simulink model "purePursuit"  (R2021b)
settings: Solver=VariableStepAuto  StartTime=0.0  StopTime=250  RelTol=1e-3
model workspace (MAT data in the model file):
  dg = 0.2
settings Model: Creator=ferna  LastModifiedBy=ferna

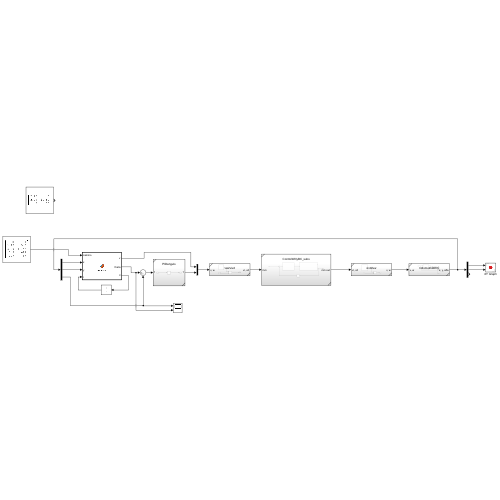
[thumbnail: Simulink's stored preview of the top-level diagram]
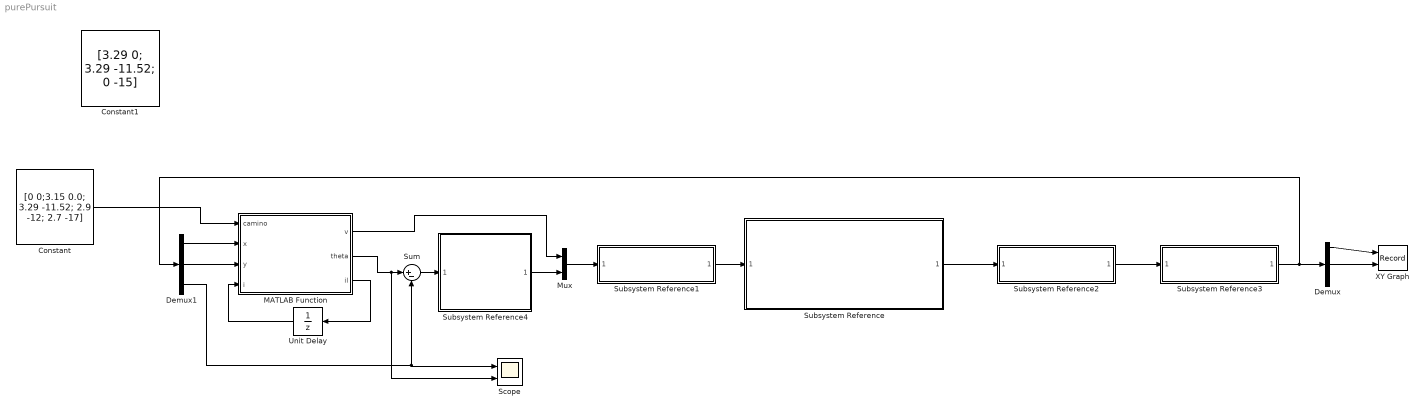
== system purePursuit ==
  Constant : Constant  Value="[0 0;3.15 0.0;  3.29 -11.52; 2.9 -12; 2.7 -17]"  SampleTime=0.01
  Constant1 : Constant  Value="[3.29 0;  3.29 -11.52; 0 -15]"  SampleTime=0.01
  Demux : Demux  Outputs=3
  Demux1 : Demux  Outputs=3
  MATLAB Function : MATLAB Function  TreatAsAtomicUnit=on
  Mux : Mux  Inputs=2
  Scope : Scope  NumInputPorts=2
  Subsystem Reference : Subsystem  ReferencedSubsystem=ControlWillyBC_subs
  Subsystem Reference1 : Subsystem  ReferencedSubsystem=vw2vivd
  Subsystem Reference2 : Subsystem  ReferencedSubsystem=vivd2vw
  Subsystem Reference3 : Subsystem  ReferencedSubsystem=OdometriaWilly
  Subsystem Reference4 : Subsystem  ReferencedSubsystem=PIDangulo
  Sum : Sum  Inputs=|+-
  Unit Delay : UnitDelay  SampleTime=-1  HasFrameUpgradeWarning=on
  XY Graph : Record  FileSettingsInternal="{\"entries\":[{\"content\":{\"excelSettings\":{\"content\":{},\"type\":\"Streamout.ExcelSettings\"}},\"type\":\"Streamout.FileSettingStorage\",\"uuid\":\"8ebd8101-3c9c-4c8a-845f-05d8ffee10d0\"}],\"packageUris\":[\"http://schema.mathworks.com/mf0/streamout_blocks/R2020a\"],\"version\":\"1.0\"}"  Layout=[1 1]  SignalsInternal="{\"entries\":[{\"content\":{\"signals\":[{\"content\":{\"blockPath\":[\"purePursuit/XY Graph\"],\"channel\":[],\"dimensions\":[1],\"domain\":\"purePursuit/XY Graph\",\"lineColor\":\"#a2142f\",\"plots\":[1],\"port\":1,\"sid\":[\"\"],\"signalID\":47498,\"signalName\":\"Demux:1\"},\"type\":\"RecordBlkView.Signal\",\"uuid\":\"32415692-7214-46dd-a3da-8b7ee7497ef6\"},{\"content\":{\"blockPath\":[\"purePursuit/XY Graph\"],\"channel\":[],\"dimensions\":[1],\"domain\":\"purePursuit/XY Graph\",\"lineColor\":\"#139fff\",\"plots\":[1],\"port\":2,\"sid\":[\"\"],\"signalID\":47502,\"signalName\":\"Demux:2\"},\"type\":\"RecordBlkView.Signal\",\"uuid\":\"e9c51910-9b07-4659-8263-b0bdf81c70b6\"}]},\"type\":\"RecordBlkView.InputSignals\",\"uuid\":\"ef43bbf9-cefa-4f18-b3d4-8c56cded70bd\"}],\"packageUris\":[\"http://schema.mathworks.com/mf0/streamout_blocks/R2020a\"],\"version\":\"1.0\"}"  VisualizationBindings="{\"xyplotplugin\":{\"info\":[{\"series\":[{\"bindingParametersList\":[{\"parameter\":\"X-Axis\",\"signalID\":47498,\"signalName\":\"Demux:1\"},{\"parameter\":\"Y-Axis\",\"signalID\":47502,\"signalName\":\"Demux:2\"}],\"seriesID\":31998}],\"subplotID\":1}]}}"  CompatibilityTag=XY
  wires:
  Demux/2 -> XY Graph/2
  MATLAB Function/2(theta) -> Scope/2, Sum/1
  Demux/1 -> XY Graph/1
  Subsystem Reference/1 -> Subsystem Reference2/1
  Subsystem Reference1/1 -> Subsystem Reference/1
  Subsystem Reference3/1 -> Demux1/1, Demux/1
  Subsystem Reference2/1 -> Subsystem Reference3/1
  MATLAB Function/1(v) -> Mux/1
  Sum/1 -> Subsystem Reference4/1
  Demux1/2 -> MATLAB Function/3(y)
  Mux/1 -> Subsystem Reference1/1
  Demux1/1 -> MATLAB Function/2(x)
  Subsystem Reference4/1 -> Mux/2
  Demux1/3 -> Sum/2, Scope/1
  MATLAB Function/3(il) -> Unit Delay/1
  Unit Delay/1 -> MATLAB Function/4(i)
  Constant/1 -> MATLAB Function/1(camino)

== matlab function purePursuit/MATLAB Function ==
  data: camino input; v output; x input; y input; i input; theta output; il output
function [v, theta, il] = posicion (camino, x, y, i)

    %Inicializamos variables de salida
    
    L=0.12; % distancia de persecucion
    v=0.3;
    i=i+1;
    
    if length(camino) >= i % mientras haya camino
    
        % Calculamos distancia al objetivo
    
        distancia=sqrt((camino(i,1) -x)^2 + (camino(i,2)-y)^2);
        
        while ((distancia < L) && (length(camino) > i)) % ya hemos llegado 
            i=i+1; % actualizar el objetivo 
            distancia = sqrt((camino (i,1) -x)^2 + (camino (i, 2) -y)^2);
            v=0.15;
        end
    
        %Calculo de la orientacion al punto i-esimo 
        theta = atan2((camino (i,2)-y), (camino (i, 1) -x));

    else % si se ha llegado al final del camino

        theta = 0;
        v = 0;
    
    end

    if i < length(camino)
        il = i - 1;
    else
        il=i;
    end


end
